simulink model "bt2_arm"  (R2019a)
settings: Solver=ode5  StartTime=0.0  StopTime=60  FixedStep=0.01  RelTol=1e-3
model workspace (MAT data in the model file):
  k0 = Simulink.Parameter
  k0.DataType = 'auto'
  k0.Dimensions = [0 0]
undefined symbols (not defined in the file): sigbuilder_block
libraries: fuzblock x1
settings Model: Creator=ASUS  LastModifiedBy=ASUS

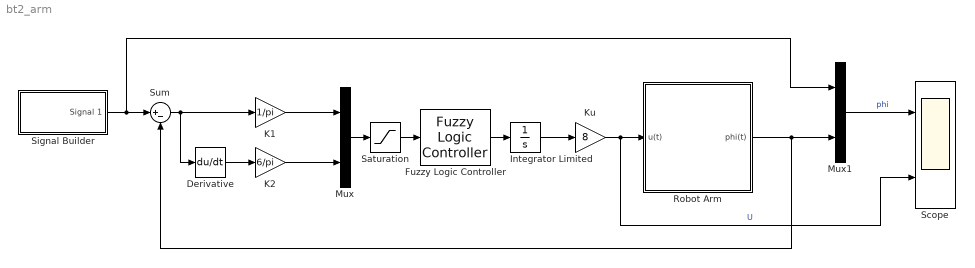
== system bt2_arm ==
  Derivative : Derivative
  Fuzzy Logic Controller : fuzblock/Fuzzy Logic  Controller  FIS='bt2.fis'  OutputSampleNumber=101  DataType=double  FuzzifiedInputs=off  RuleFiringStrengths=off  RuleOutputs=off  AggregatedOutputs=off  SimulateUsing=Interpreted execution  OutOfRangeInputValueMessage=warning  NoRuleFiredMessage=warning  EmptyOutputFuzzySetMessage=warning
  Integrator Limited : Integrator  LimitOutput=on  UpperSaturationLimit=1  LowerSaturationLimit=-1
  K1 : Gain  Gain=1/pi
  K2 : Gain  Gain=6/pi
  Ku : Gain  Gain=8
  Mux : Mux  Inputs=2
  Mux1 : Mux  Inputs=2
  Robot Arm : Subsystem  mask{M=1, m_=0.1, l=0.4, lc=0.15, B=0.2, g=9.81, J=0.05}
  Saturation : Saturate  UpperLimit=1  LowerLimit=-1
  Scope : Scope  NumInputPorts=2
  Signal Builder : Subsystem  Tag=STV Subsys  LoadFcn=sigbuilder_block('load');  StartFcn=sigbuilder_block('start');  StopFcn=sigbuilder_block('stop');  ClipboardFcn=sigbuilder_block('clipboard');  mask(Sigbuilder block){tuvar=[0:10]}
      mask help: Simulink:masks:SigbuilderBlock_MD
      mask init:
      | if ~strcmp(get_param(bdroot(gcbh),'SimulationStatus'),'stopped') tuvar = sigbuilder_block('maskInit'); end
      settings: CopyFcn=sigbuilder_block('copy');  DeleteFcn=sigbuilder_block('delete');  ModelCloseFcn=sigbuilder_block('modelClose');  PreSaveFcn=sigbuilder_block('preSave');  PauseFcn=sigbuilder_block('pause');  ContinueFcn=sigbuilder_block('continue');  NameChangeFcn=sigbuilder_block('namechange');  OpenFcn=sigbuilder_block('open',[538.8 144.6 550.8 400.2 ]);  CloseFcn=sigbuilder_block('close');
      mask Display: plot(0, 0, 100, 100,[2, 2, 32, 32, 2], [68, 8, 8, 68, 68],[32, 2], [38, 38], [32, 19, 2],[53, 60, 44], [32, 17, 17, 2],[16, 16, 31, 31]);txt = getActiveGroup(gcbh);text(2, 100, txt,'verticalAlignment', 'top');
  Sum : Sum  Inputs=|+-
  wires:
  Ku/1 -> Scope/2, Robot Arm/1(u(t))  "U"
  Saturation/1 -> Fuzzy Logic Controller/1
  Mux/1 -> Saturation/1
  Derivative/1 -> K2/1
  Sum/1 -> K1/1, Derivative/1
  K1/1 -> Mux/1
  K2/1 -> Mux/2
  Signal Builder/1(Signal 1) -> Mux1/1, Sum/1
  Robot Arm/1(phi(t)) -> Sum/2, Mux1/2
  Mux1/1 -> Scope/1  "phi"
  Fuzzy Logic Controller/1 -> Integrator Limited/1
  Integrator Limited/1 -> Ku/1

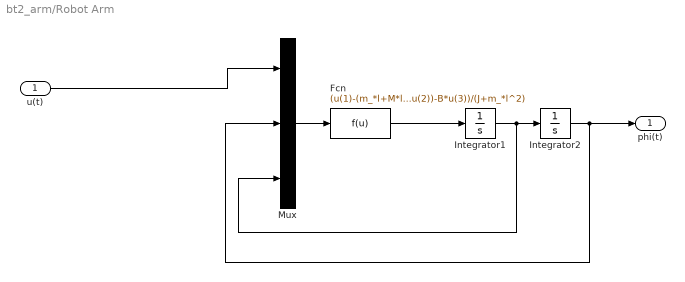
== system bt2_arm/Robot Arm ==
  u(t) : Inport
  Fcn : Fcn  Expr=(u(1)-(m_*l+M*lc)*g*sin(u(2))-B*u(3))/(J+m_*l^2)
  Integrator1 : Integrator
  Integrator2 : Integrator
  Mux : Mux  Inputs=3
  phi(t) : Outport
  wires:
  Integrator1/1 -> Mux/3, Integrator2/1
  Integrator2/1 -> Mux/2, phi(t)/1
  Mux/1 -> Fcn/1
  u(t)/1 -> Mux/1
  Fcn/1 -> Integrator1/1

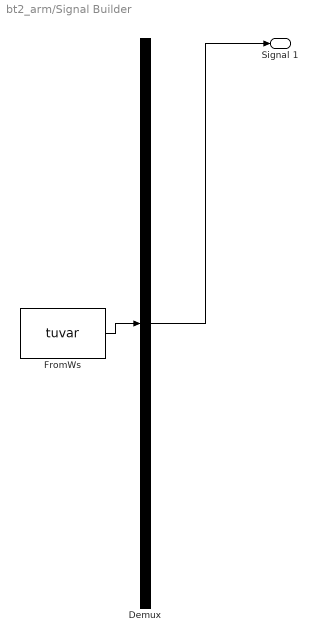
== system bt2_arm/Signal Builder ==
  Demux : Demux  Tag=STV Demux  Outputs=1
  FromWs : FromWorkspace  Tag=STV FromWs  VariableName=tuvar  SampleTime=0
      SigBuilderData=|
      | common.afterFinalStr = 'Extrapolate'
      | common.sampleTime = 0
      | dataSet.timeRange = [0 60]
      | dataSet.name = 'Group 1'
      | sbobj.Groups.Name = 'Group 1'
      | sbobj.Groups.Signals.Name = 'Signal 1'
      | sbobj.Groups.Signals.XData = [0 14.4 14.4 29.7 29.7 45 45 60]
      | sbobj.Groups.Signals.YData = [2.27 2.27 1.15 1.15 1.74 1.74 0.22 0.22]
      | sbobj.Groups.TimeRange = [0 60]
  Signal 1 : Outport  Tag=STV Outport
  wires:
  Demux/1 -> Signal 1/1
  FromWs/1 -> Demux/1
